simulink subsystem "rss_EcuGateChargeCircuit"  (R2022b)
settings: Solver=VariableStepAuto  StartTime=0.0  StopTime=10.0  RelTol=1e-3
undefined symbols (not defined in the file): cstChrgCrctPrllRstn, cstGateRstn
libraries: fl_lib x3, ee_lib x1
settings Model: Creator=CAV2OFO  LastModifiedBy=CAV2OFO

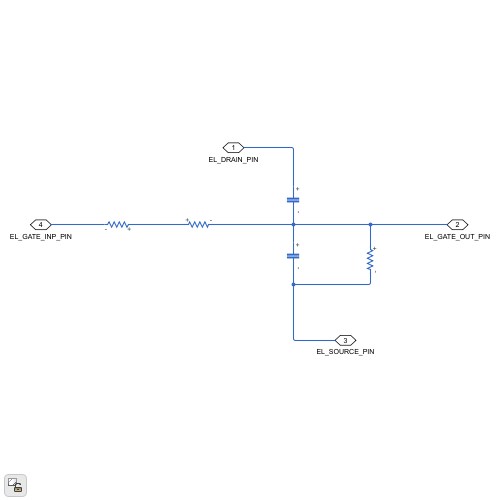
[thumbnail: Simulink's stored preview of the top-level diagram]
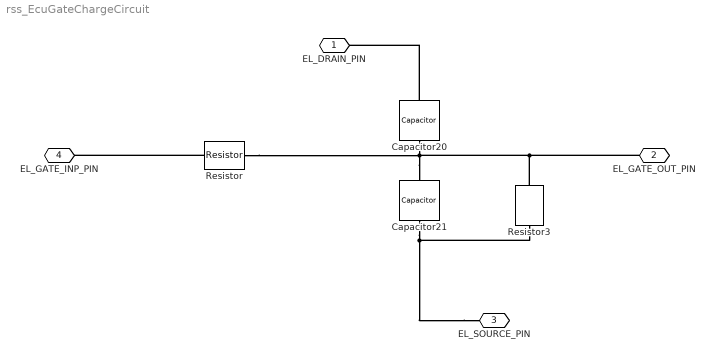
== system rss_EcuGateChargeCircuit ==
  Capacitor20 : fl_lib/Electrical/Electrical Elements/Capacitor  c=cstChrgCrctSrsCpct F  r=cstChrgCrctSrsCpcrRstn Ohm  g=0 1/Ohm  i_specify=off  i_priority=None  i=0 A  i_nominal_specify=off  i_nominal_unit=A  i_nominal_value=1  v_specify=off  v_priority=None  v=0 V  v_nominal_specify=off  v_nominal_unit=V  v_nominal_value=1  vc_specify=off  vc_priority=High  vc=0 V  vc_nominal_specify=off  vc_nominal_unit=V  vc_nominal_value=1
  Capacitor21 : fl_lib/Electrical/Electrical Elements/Capacitor  c=cstChrgCrctPrllCpct F  r=cstChrgCrctPrllCpcrRstn Ohm  g=0 1/Ohm  i_specify=off  i_priority=None  i=0 A  i_nominal_specify=off  i_nominal_unit=A  i_nominal_value=1  v_specify=off  v_priority=High  v=0 V  v_nominal_specify=off  v_nominal_unit=V  v_nominal_value=1  vc_specify=off  vc_priority=High  vc=12 V  vc_nominal_specify=off  vc_nominal_unit=V  vc_nominal_value=1
  Resistor : ee_lib/Passive/Resistor  R=cstGateRstn Ohm  enable_R_tol=0  R_tol=5  tol_distribution=1  nSigma=4  enable_operating_limits=0  operating_limit_action=2  max_working_voltage=100 V  power_rating=1 W  enable_faults=0  fault_action=1  R_faulted=inf Ohm  enable_temporal_fault=0  t_fault=1 s  enable_behavioral_fault=0  max_permissible_current=1 A  t_fail_on_current=1 s  noise_mode=0  sample_time=1e-3 s  repeatability=1  auto_seed=1370255919  user_seed=0  Tdevice=25 degC  power_derating_T1=70 degC  power_derating_T2=155 degC  operating_temperature_range_vec=[-50, 150] degC  alpha=3.93e-3 1/K  Tmeas=25 degC  thermal_mass=100 J/K  temperature_specify=off  temperature_priority=High  temperature=298.15 K  temperature_nominal_specify=off  temperature_nominal_unit=K  temperature_nominal_value=1
  Resistor3 : fl_lib/Electrical/Electrical Elements/Resistor  R=cstChrgCrctPrllRstn Ohm  i_specify=off  i_priority=None  i=0 A  i_nominal_specify=off  i_nominal_unit=A  i_nominal_value=1  v_specify=off  v_priority=None  v=0 V  v_nominal_specify=off  v_nominal_unit=V  v_nominal_value=1
  EL_DRAIN_PIN : PMIOPort  Side=Left
  EL_GATE_OUT_PIN : PMIOPort  Port=2  Side=Right
  EL_SOURCE_PIN : PMIOPort  Port=3  Side=Right
  EL_GATE_INP_PIN : PMIOPort  Port=4  Side=Left
  connections:
  Capacitor21/LConn1 -- EL_GATE_OUT_PIN/RConn1 -- Resistor3/LConn1 -- Resistor/RConn1 -- Capacitor20/RConn1
  EL_SOURCE_PIN/RConn1 -- Capacitor21/RConn1 -- Resistor3/RConn1
  Resistor/LConn1 -- EL_GATE_INP_PIN/RConn1
  Capacitor20/LConn1 -- EL_DRAIN_PIN/RConn1
